simulink model "complex_UIO"  (R2019b)
settings: Solver=VariableStepAuto  StartTime=0.0  StopTime=10.0  RelTol=1e-3
values from neighbouring files (symbols this model uses):
  Ac = [real(A) -imag(A);imag(A) real(A)]    [DAC_UIO_Comp.m]    (also in LinearND_QUANTUM_2020_11_14_2.m = [realA -imagA;imagA realA]; UIO_alternative_2021_01_26.m; UIO_alternative_PAPER_2021_02_17.m = Abar(2:3,2:3); UIO_alternative_PAPER_2021_03_01.m = Abar(2:3,2:3))
  Am = double(subs(Am_sys,{ep,Lx},{0.1,1-2*j}))    [DAC_UIO_Comp.m]    (also in UIO_adaptive_example_EEG_Balas_2ch.m = [0 1;-5 -4]; UIO_adaptive_example_alternative_EEG_ch6.m = ss_c.A; UIO_alternative_2021_01_26.m = Am-.1*eye(2); UIO_alternative_PAPER_2021_02_17.m = [0 1;-1 -1])
  Amc = [real(Am) -imag(Am);imag(Am) real(Am)]    [DAC_UIO_Comp.m]    (also in UIO_alternative_2021_01_26.m)
  B = [0;1]    [DAC_UIO_Comp.m]    (also in UIO_adaptive_example_EEG_Balas_2ch.m; UIO_adaptive_example_alternative_EEG_ch6.m = ones(opt_order,1); UIO_alternative_2021_01_26.m; UIO_alternative_PAPER_2021_02_17.m = [1;0;-1])
  Bc = [real(B) -imag(B);imag(B) real(B)]    [DAC_UIO_Comp.m]    (also in UIO_alternative_2021_01_26.m; UIO_alternative_PAPER_2021_02_17.m = Bbar(2:3,:); UIO_alternative_PAPER_2021_03_01.m = Bbar(2:3,:))
  C = double(subs(C_sym,{ep},{0.1}))    [DAC_UIO_Comp.m]    (also in UIO_adaptive_example.m = [1 0 0 0 0;0 0 0 1 0; 0 0 0 0 1]; UIO_adaptive_example_2.m = [1 0 0 0;0 1 0 0]; UIO_adaptive_example_EEG_Balas_2ch.m = [1, epsilon]; UIO_adaptive_example_alternative_EEG_ch6.m = ss_c.C)
  g1 = 4+2j    [DAC_UIO_Comp.m]    (also in UIO_adaptive_example_EEG_Balas_2ch.m = 4; UIO_alternative_2021_01_26.m = 2+1j; UIO_alternative_PAPER_2021_02_17.m = 2; UIO_alternative_PAPER_2021_03_01.m = 2)
  g2 = 0    [DAC_UIO_Comp.m]    (also in UIO_adaptive_example_EEG_Balas_2ch.m = -0.3; UIO_alternative_2021_01_26.m; UIO_alternative_PAPER_2021_02_17.m = 1; UIO_alternative_PAPER_2021_03_01.m)
  g3 = 0    [DAC_UIO_Comp.m]    (also in UIO_adaptive_example_EEG_Balas_2ch.m = 0.1; UIO_alternative_2021_01_26.m; UIO_alternative_PAPER_2021_02_17.m = -3; UIO_alternative_PAPER_2021_03_01.m)
  gamma_e = 1    [DAC_UIO_Comp.m]    (also in UIO_adaptive_example_EEG_Balas_2ch.m; UIO_adaptive_example_alternative_EEG_ch6.m = .0001*ones(length(Am),1); UIO_alternative_2021_01_26.m = 0.001; UIO_alternative_PAPER_2021_02_17.m = 0.0001)
  gamma_u = 1    [DAC_UIO_Comp.m]    (also in UIO_adaptive_example_EEG_Balas_2ch.m = 2)
settings Model: Creator=Tris  LastModifiedBy=Tris

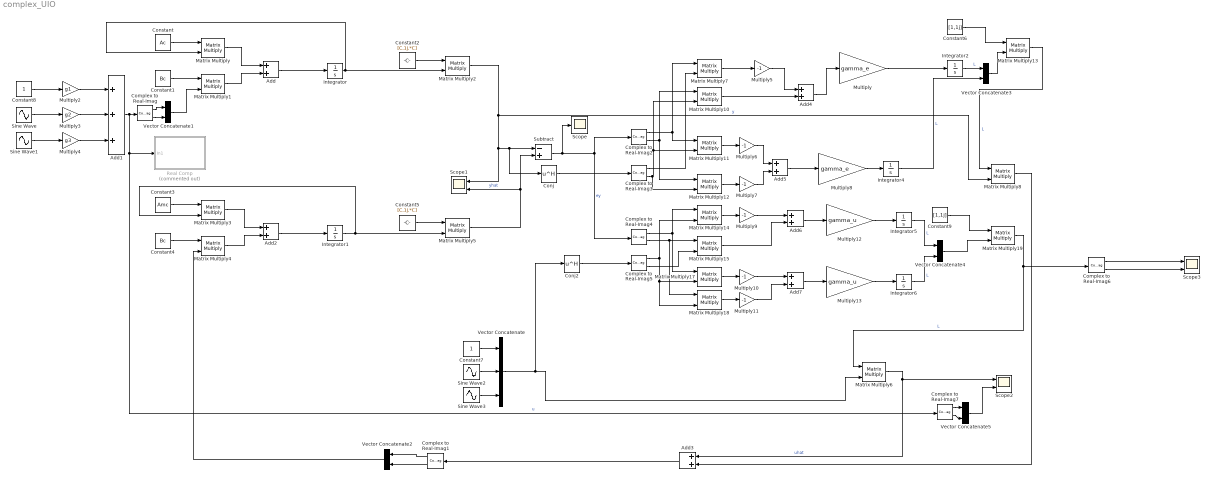
== system complex_UIO ==
  Add{,2..7} (7 alike) : Sum
  Add1 : Sum  Inputs=+++
  Complex to Real-Imag{,1..7} (8 alike) : ComplexToRealImag
  Conj : Math  Operator=hermitian  SignedPower=off  SaturateOnIntegerOverflow=on
  Conj2 : Math  Operator=hermitian  SignedPower=off  SaturateOnIntegerOverflow=on
  Constant : Constant  Value=Ac
  Constant1 : Constant  Value=Bc  VectorParams1D=off
  Constant2 : Constant  Value=[C,1j.*C]  VectorParams1D=off
  Constant3 : Constant  Value=Amc
  Constant4 : Constant  Value=Bc  VectorParams1D=off
  Constant5 : Constant  Value=[C,1j.*C]  VectorParams1D=off
  Constant6 : Constant  Value=[1,1j]  VectorParams1D=off
  Constant7 : Constant  VectorParams1D=off
  Constant8 : Constant  VectorParams1D=off
  Constant9 : Constant  Value=[1,1j]  VectorParams1D=off
  Integrator{,1..2,4..6} (6 alike) : Integrator
  Matrix Multiply{,1..8,10..15,17..19} (18 alike) : Product  Multiplication=Matrix(*)
  Multiply : Gain  Gain=gamma_e
  Multiply{5..7,9..11} (6 alike) : Gain  Gain=-1
  Multiply12 : Gain  Gain=gamma_u
  Multiply13 : Gain  Gain=gamma_u
  Multiply2 : Gain  Gain=g1
  Multiply3 : Gain  Gain=g2
  Multiply4 : Gain  Gain=g3
  Multiply8 : Gain  Gain=gamma_e
  Real Comp : Subsystem  Commented=on
  Scope : Scope
  Scope1 : Scope  NumInputPorts=2
  Scope2 : Scope  NumInputPorts=2
  Scope3 : Scope  NumInputPorts=2
  Sine Wave : Sin  SampleTime=0  VectorParams1D=off
  Sine Wave1 : Sin  Phase=pi/2  SampleTime=0  VectorParams1D=off
  Sine Wave2 : Sin  SampleTime=0  VectorParams1D=off
  Sine Wave3 : Sin  Phase=pi/2  SampleTime=0  VectorParams1D=off
  Subtract : Sum  Inputs=-+
  Vector Concatenate : Concatenate  NumInputs=3  Mode=Multidimensional array
  Vector Concatenate{1..5} (5 alike) : Concatenate  Mode=Multidimensional array
  wires:
  Constant/1 -> Matrix Multiply/1
  Integrator/1 -> Matrix Multiply2/2, Matrix Multiply/2
  Add/1 -> Integrator/1
  Matrix Multiply/1 -> Add/1
  Matrix Multiply1/1 -> Add/2
  Constant1/1 -> Matrix Multiply1/1
  Multiply4/1 -> Add1/3
  Multiply3/1 -> Add1/2
  Multiply2/1 -> Add1/1
  Sine Wave1/1 -> Multiply4/1
  Constant8/1 -> Multiply2/1
  Sine Wave/1 -> Multiply3/1
  Constant2/1 -> Matrix Multiply2/1
  Matrix Multiply2/1 -> Matrix Multiply8/2, Conj/1, Subtract/1, Scope1/1  "y"
  Add1/1 -> Complex to Real-Imag7/1, Real Comp/1(In1), Complex to Real-Imag/1  "u"
  Constant3/1 -> Matrix Multiply3/1
  Constant4/1 -> Matrix Multiply4/1
  Matrix Multiply4/1 -> Add2/2
  Matrix Multiply3/1 -> Add2/1
  Add2/1 -> Integrator1/1
  Integrator1/1 -> Matrix Multiply5/2, Matrix Multiply3/2
  Constant5/1 -> Matrix Multiply5/1
  Matrix Multiply5/1 -> Subtract/2, Scope1/2  "yhat"
  Multiply/1 -> Integrator2/1
  Subtract/1 -> Scope/1, Complex to Real-Imag4/1, Complex to Real-Imag2/1  "ey"
  Sine Wave2/1 -> Vector Concatenate/2
  Constant7/1 -> Vector Concatenate/1
  Sine Wave3/1 -> Vector Concatenate/3
  Vector Concatenate/1 -> Conj2/1, Matrix Multiply6/2
  Matrix Multiply6/1 -> Add3/1, Scope2/1  "uhat"
  Matrix Multiply8/1 -> Add3/2
  Complex to Real-Imag/1 -> Vector Concatenate1/1
  Complex to Real-Imag/2 -> Vector Concatenate1/2
  Vector Concatenate1/1 -> Matrix Multiply1/2
  Add3/1 -> Complex to Real-Imag1/1
  Complex to Real-Imag1/2 -> Vector Concatenate2/2
  Complex to Real-Imag1/1 -> Vector Concatenate2/1
  Vector Concatenate2/1 -> Matrix Multiply4/2
  Complex to Real-Imag2/1 -> Matrix Multiply11/1, Matrix Multiply7/1
  Conj/1 -> Complex to Real-Imag3/1
  Complex to Real-Imag3/1 -> Matrix Multiply7/2
  Matrix Multiply7/1 -> Multiply5/1
  Matrix Multiply10/1 -> Add4/2
  Add4/1 -> Multiply/1
  Complex to Real-Imag2/2 -> Matrix Multiply10/1, Matrix Multiply12/1
  Complex to Real-Imag3/2 -> Matrix Multiply12/2, Matrix Multiply11/2, Matrix Multiply10/2
  Multiply5/1 -> Add4/1
  Matrix Multiply11/1 -> Multiply6/1
  Matrix Multiply12/1 -> Multiply7/1
  Multiply6/1 -> Add5/1
  Multiply7/1 -> Add5/2
  Add5/1 -> Multiply8/1
  Multiply8/1 -> Integrator4/1
  Integrator2/1 -> Vector Concatenate3/1  "L"
  Integrator4/1 -> Vector Concatenate3/2  "L"
  Vector Concatenate3/1 -> Matrix Multiply13/2
  Constant6/1 -> Matrix Multiply13/1
  Matrix Multiply13/1 -> Matrix Multiply8/1  "L"
  Complex to Real-Imag4/1 -> Matrix Multiply14/1, Matrix Multiply17/1
  Complex to Real-Imag5/1 -> Matrix Multiply14/2, Matrix Multiply18/2, Matrix Multiply17/2
  Complex to Real-Imag4/2 -> Matrix Multiply18/1, Matrix Multiply15/1
  Complex to Real-Imag5/2 -> Matrix Multiply15/2
  Matrix Multiply14/1 -> Multiply9/1
  Matrix Multiply17/1 -> Multiply10/1
  Matrix Multiply18/1 -> Multiply11/1
  Multiply9/1 -> Add6/1
  Matrix Multiply15/1 -> Add6/2
  Multiply10/1 -> Add7/1
  Multiply11/1 -> Add7/2
  Add6/1 -> Multiply12/1
  Add7/1 -> Multiply13/1
  Multiply12/1 -> Integrator5/1
  Multiply13/1 -> Integrator6/1
  Integrator5/1 -> Vector Concatenate4/1  "L"
  Integrator6/1 -> Vector Concatenate4/2  "L"
  Constant9/1 -> Matrix Multiply19/1
  Vector Concatenate4/1 -> Matrix Multiply19/2
  Conj2/1 -> Complex to Real-Imag5/1
  Matrix Multiply19/1 -> Complex to Real-Imag6/1, Matrix Multiply6/1  "L"
  Complex to Real-Imag6/1 -> Scope3/1
  Complex to Real-Imag6/2 -> Scope3/2
  Complex to Real-Imag7/1 -> Vector Concatenate5/1
  Complex to Real-Imag7/2 -> Vector Concatenate5/2
  Vector Concatenate5/1 -> Scope2/2

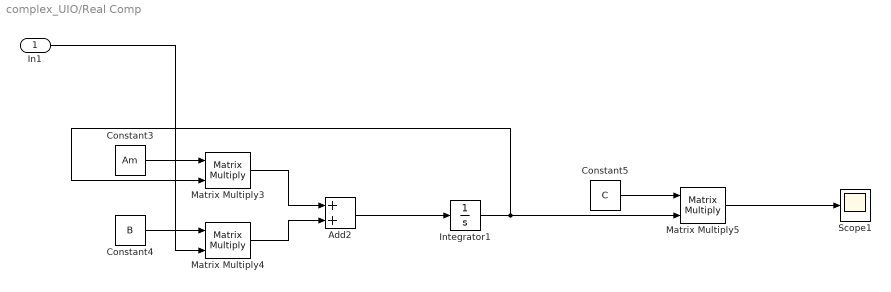
== system complex_UIO/Real Comp ==
  In1 : Inport
  Add2 : Sum
  Constant3 : Constant  Value=Am
  Constant4 : Constant  Value=B  VectorParams1D=off
  Constant5 : Constant  Value=C  VectorParams1D=off
  Integrator1 : Integrator
  Matrix Multiply3 : Product  Multiplication=Matrix(*)
  Matrix Multiply4 : Product  Multiplication=Matrix(*)
  Matrix Multiply5 : Product  Multiplication=Matrix(*)
  Scope1 : Scope
  wires:
  Constant5/1 -> Matrix Multiply5/1
  Integrator1/1 -> Matrix Multiply3/2, Matrix Multiply5/2
  Matrix Multiply4/1 -> Add2/2
  Constant4/1 -> Matrix Multiply4/1
  Add2/1 -> Integrator1/1
  Matrix Multiply5/1 -> Scope1/1
  In1/1 -> Matrix Multiply4/2
  Constant3/1 -> Matrix Multiply3/1
  Matrix Multiply3/1 -> Add2/1
